simulink model "MicroMouseTemplate"  (R2024a)
settings: Solver=FixedStepAuto  StartTime=0.0  StopTime=10.0  RelTol=1e-3  EnableMultiTasking=on
undefined symbols (not defined in the file): DownLSThreshConv, DownRSThreshConv, FWDLSThreshConv, FWDRSThreshConv, LSThreshConv, RSThreshConv, samplingTime
settings Model: STM32="{\"DigitalPortWrite\":[{\"ID\":\"MicroMouseTemplate:84:10\"},{\"ID\":\"MicroMouseTemplate:84:9\"},{\"ID\":\"MicroMouseTemplate:84:8\"},{\"ID\":\"MicroMouseTemplate:84:7\"},{\"ID\":\"MicroMouseTemplate:84:6\"},{\"ID\":\"MicroMouseTemplate:84:5\"},{\"ID\":\"MicroMouseTemplate:84:4\"},{\"ID\":\"MicroMouseTemplate:84:3\"},{\"ID\":\"MicroMouseTemplate:160:19\"},{\"ID\":\"MicroMouseTemplate:2479:4\"},{\"ID\":\"MicroMouseTemplate:2479:6\"},{\"ID\":\"MicroMouseTemplate:2479:7\"},{\"ID\":\"MicroMouseTemplate:2479:8\"}],\"PWMOutput\":[{\"ID\":\"MicroMouseTemplate:160:24\"},{\"ID\":\"MicroMouseTemplate:160:25\"}],\"AnalogInput\":{\"ID\":\"MicroMouseTemplate:2357:1\"},\"DigitalPortRead\":[{\"ID\":\"MicroMouseTemplate:2483:3\"},{\"ID\":\"MicroMouseTemplate:2483:4\"}]}"  SimulationMode=external  ExtModeTrigDuration=10  Creator=JesseJabezArendse  LastModifiedBy=abdul
settings SolverCC: AllowMultiTaskInputOutput=on  AutoInsertRateTranBlk=on  InsertRTBMode=Never (minimum delay)
settings OptimizationCC: EnhancedBackFolding=on  PassReuseOutputArgsAs=Individual arguments  StateBitsets=on  DataBitsets=on  ZeroExternalMemoryAtStartup=off  ZeroInternalMemoryAtStartup=off  NoFixptDivByZeroProtection=on  MaxStackSize=64  OptimizeBlockOrder=speed  DifferentSizesBufferReuse=on  EfficientTunableParamExpr=on
settings DebuggingCC: MultiTaskCondExecSysMsg=none  ParameterOverflowMsg=none  ParameterPrecisionLossMsg=none  ParameterTunabilityLossMsg=error
settings HardwareCC: ProdBitPerPointer=32  ProdBitPerSizeT=32  ProdBitPerPtrDiffT=32  ProdLargestAtomicInteger=Long  ProdLargestAtomicFloat=Double  ProdWordSize=32  ProdLongLongMode=on  ProdHWDeviceType=ARM Compatible->ARM Cortex  TargetBitPerPointer=64  TargetBitPerSizeT=64  TargetBitPerPtrDiffT=64  TargetLongLongMode=on  TargetIntDivRoundTo=Zero  TargetEndianess=LittleEndian  TargetWordSize=64  TargetHWDeviceType=MATLAB Host
settings ModelReferenceCC: EnableParallelModelReferenceBuilds=on  ParallelModelReferenceMATLABWorkerInit=Copy Base Workspace  SupportModelReferenceSimTargetCustomCode=on
settings SFSimCC: MATLABDynamicMemAlloc=off  SimHardwareAcceleration=native
settings RTWCC: Description=Embedded Coder  SystemTargetFile=ert.tlc  HardwareBoard=STM32L4xx Based  TLCOptions=-p0 -aInlineSetEventsForThisBaseRateFcn=TLC_FALSE -aSuppressMultiTaskScheduler=TLC_FALSE -aRateBasedStepFcn=1  TemplateMakefile=ert_default_tmf  Toolchain=GNU Tools for ARM Embedded Processors  CodeExecutionProfiling=on  CodeProfilingInstrumentation=coarse  GPUComputeCapability=3.5
settings RTWCC: CustomHeaderCode=|
  | #include "MicroMouseProgramming\Core\Inc\IMU.h"
  | #include "MicroMouseProgramming\Core\Inc\CustomWhile.h"
  | #include "MicroMouseProgramming\Core\Inc\Motors.h"
settings RTWCC: CustomInclude=|
  | MicroMouseProgramming\Core\Inc\
  | MicroMouseProgramming\Core\Src\
settings RTWCC: CustomSource=|
  | MicroMouseProgramming\Core\Src\IMU.c
  | MicroMouseProgramming\Core\Src\CustomWhile.c
  | MicroMouseProgramming\Core\Src\Motors.c
settings CodeAppCC: ForceParamTrailComments=on  IgnoreCustomStorageClasses=off  OperatorAnnotations=on  SimulinkDataObjDesc=on  SFDataObjDesc=on  InsertBlockDesc=on
settings ERTTargetCC: CodeReplacementLibrary=ARM Cortex-M  SupportNonFinite=off  SupportComplex=off  SupportContinuousTime=on  ExtModeTransport=3  ExtModeStaticAlloc=on  ExtModeStaticAllocSize=2048  ExtModeMexFile=ext_xcp  ExtModeIntrfLevel=Level2 - Open

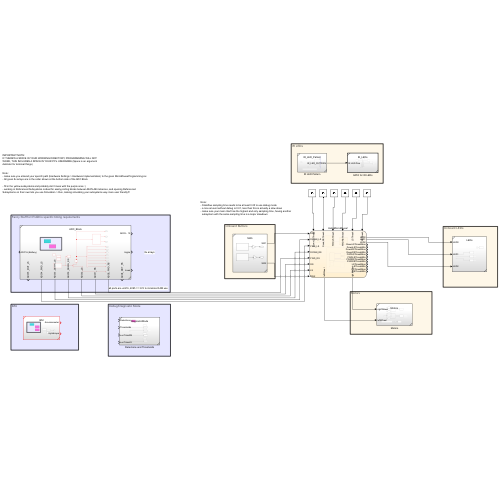
[thumbnail: Simulink's stored preview of the top-level diagram]
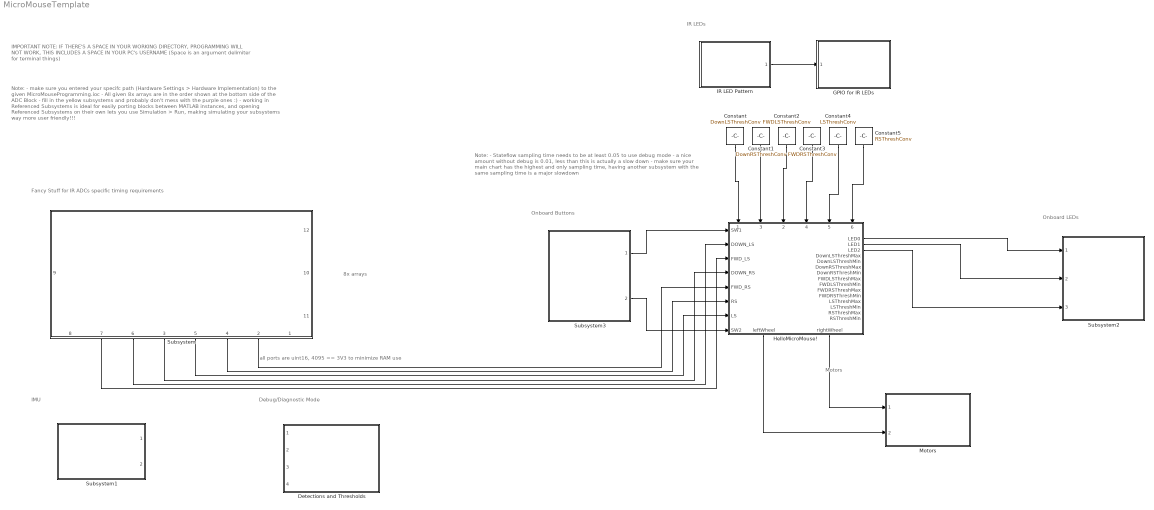
== system MicroMouseTemplate ==
  note: IMPORTANT NOTE:
      | IF THERE'S A SPACE IN YOUR WORKING DIRECTORY, PROGRAMMING WILL NOT WORK, THIS INCLUDES A SPACE IN YOUR PC's USERNAME (Space is an argument delimiter for terminal things)
  note: Note:
      | - make sure you entered your specifc path (Hardware Settings > Hardware Implementation) to the given MicroMouseProgramming.ioc
      | - All given 8x arrays are in the order shown at the bottom side of the ADC Block
      |
      | - fill in the yellow subsystems and probably don't mess with the purple ones :)
      | - working in Referenced Subsystems is ideal for easily porting blocks between MATLAB instances, and opening Referenced Subsystems on their own lets you use Simulation > Run, making simulating your subsystems way more user friendly!!!
  note: 8x arrays
  note: all ports are uint16, 4095 == 3V3 to minimize RAM use
  note: IMU
  note: Note:
      | - Stateflow sampling time needs to be at least 0.05 to use debug mode
      | - a nice amount without debug is 0.01, less than this is actually a slow down
      | - make sure your main chart has the highest and only sampling time, having another
      | subsystem with the same sampling time is a major slowdown
  note: Fancy Stuff for IR ADCs specific timing requirements
  note: IR LEDs
  note: Motors
  note: Onboard Buttons
  note: Onboard LEDs
  note: Debug/Diagnostic Mode
  Constant : Constant  Value=DownLSThreshConv
  Constant1 : Constant  Value=DownRSThreshConv
  Constant2 : Constant  Value=FWDLSThreshConv
  Constant3 : Constant  Value=FWDRSThreshConv
  Constant4 : Constant  Value=LSThreshConv
  Constant5 : Constant  Value=RSThreshConv
  Detections and Thresholds : Subsystem  ReferencedSubsystem=DiagnosticMode
  GPIO for IR LEDs : Subsystem  TreatAsAtomicUnit=on  SystemSampleTime=samplingTime  ReferencedSubsystem=IR_LEDs
  HelloMicroMouse! : Stateflow chart  TreatAsAtomicUnit=on
      settings: PortSchema="{\"entries\":[{\"content\":{\"sides\":[{\"content\":{\"connectorIds\":[\"In8\",\"In14\",\"In9\",\"In10\",\"In11\",\"In12\",\"In13\",\"In7\"]},\"type\":\"ConnectorPlacement.EquallySpacedRectSide\",\"uuid\":\"f52daa4f-6374-42e5-9ef1-0ccc99d09b58\"},{\"content\":{\"connectorIds\":[\"Out4\",\"Out1\",\"Out5\",\"Out6\",\"Out7\",\"Out8\",\"Out9\",\"Out10\",\"Out11\",\"Out12\",\"Out13\",\"Out14\",\"Out15\",\"Out16\",\"Out17\"],\"side\":\"RIGHT\"},\"type\":\"ConnectorPlacement.EquallySpacedRectSide\",\"uuid\":\"94b478cc-4dde-45c7-a588-77cf2b43cdb7\"},{\"content\":{\"connectorIds\":[\"In1\",\"In3\",\"In2\",\"In4\",\"In5\",\"In6\"],\"side\":\"TOP\"},\"type\":\"ConnectorPlacement.EquallySpacedRectSide\",\"uuid\":\"afff2079-ea5c-423e-9722-09c3bbce433b\"},{\"content\":{\"connectorIds\":[\"Out2\",\"Out3\"],\"side\":\"BOTTOM\"},\"type\":\"ConnectorPlacement.EquallySpacedRectSide\",\"uuid\":\"94e93a1d-795d-41a3-b2d8-d520b2bf47ef\"}]},\"type\":\"ConnectorPlacement.EquallySpacedConnector\",\"uuid\":\"d4d35636-54af-48ac-af70-d56caef5e090\"}],\"packageUris\":[\"http://schema.mathworks.com/mf0/Connector/R2020b\"],\"version\":\"1.0\"}"
  IR LED Pattern : Subsystem  ReferencedSubsystem=IR_LED_Pattern
  Motors : Subsystem  ReferencedSubsystem=Motors
  Subsystem : Subsystem  ReferencedSubsystem=ADC_Block
      settings: PortSchema="{\"entries\":[{\"content\":{\"sides\":[{\"content\":{},\"type\":\"ConnectorPlacement.EquallySpacedRectSide\",\"uuid\":\"be6b81d5-7a49-4e34-b35f-0c07892094fc\"},{\"content\":{\"connectorIds\":[\"Out1\",\"Out2\",\"Out4\",\"Out5\",\"Out3\",\"Out6\",\"Out7\",\"Out8\"],\"side\":\"RIGHT\"},\"type\":\"ConnectorPlacement.EquallySpacedRectSide\",\"uuid\":\"5e22590a-b7c0-4c63-8de4-8d81fd6c3849\"},{\"content\":{\"connectorIds\":[\"Out12\",\"Out10\",\"Out11\"],\"side\":\"TOP\"},\"type\":\"ConnectorPlacement.EquallySpacedRectSide\",\"uuid\":\"da97636e-cea0-4a10-8fe5-d807f9ee999f\"},{\"content\":{\"connectorIds\":[\"Out9\"],\"side\":\"BOTTOM\"},\"type\":\"ConnectorPlacement.EquallySpacedRectSide\",\"uuid\":\"a593d780-81a8-4730-a8bc-2bbf356cafe4\"}]},\"type\":\"ConnectorPlacement.EquallySpacedConnector\",\"uuid\":\"0bcac921-e51a-4437-9183-315712d0a8c2\"}],\"packageUris\":[\"http://schema.mathworks.com/mf0/Connector/R2020b\"],\"version\":\"1.0\"}"
  Subsystem1 : Subsystem  ReferencedSubsystem=IMU
  Subsystem2 : Subsystem  ReferencedSubsystem=LEDs
  Subsystem3 : Subsystem  ReferencedSubsystem=SWs
  wires:
  HelloMicroMouse!/2(leftWheel) -> Motors/2
  HelloMicroMouse!/3(rightWheel) -> Motors/1
  Subsystem3/1 -> HelloMicroMouse!/8(SW1)
  Subsystem3/2 -> HelloMicroMouse!/7(SW2)
  IR LED Pattern/1 -> GPIO for IR LEDs/1
  HelloMicroMouse!/1(LED1) -> Subsystem2/2
  HelloMicroMouse!/5(LED2) -> Subsystem2/3
  HelloMicroMouse!/4(LED0) -> Subsystem2/1
  Subsystem/6 -> HelloMicroMouse!/14(DOWN_LS)
  Constant/1 -> HelloMicroMouse!/1(DownLSThresh)
  Subsystem/3 -> HelloMicroMouse!/10(DOWN_RS)
  Subsystem/7 -> HelloMicroMouse!/9(FWD_LS)
  Subsystem/2 -> HelloMicroMouse!/11(FWD_RS)
  Subsystem/5 -> HelloMicroMouse!/13(LS)
  Subsystem/4 -> HelloMicroMouse!/12(RS)
  Constant1/1 -> HelloMicroMouse!/3(DownRSThresh)
  Constant2/1 -> HelloMicroMouse!/2(FWDLSThresh)
  Constant3/1 -> HelloMicroMouse!/4(FWDRSThresh)
  Constant4/1 -> HelloMicroMouse!/5(LSThresh)
  Constant5/1 -> HelloMicroMouse!/6(RSThresh)

== stateflow chart MicroMouseTemplate/HelloMicroMouse! ==
  state Calibration
    %--------------------
    entry:
    LED1 = true;
    rightWheel = 75;
    leftWheel = -75;
    % Meausure min/max voltage received
    DownLSThreshMin = DOWN_LS;
    DownRSThreshMin = DOWN_RS;
    FWDLSThreshMin = FWD_LS;
    FWDRSThreshMin = FWD_RS;
    LSThreshMin = LS;
    RSThreshMin = RS;
    DownLSThreshMax = DOWN_LS;
    DownRSThreshMax = DOWN_RS;
    FWDLSThreshMax = FWD_LS;
    FWDRSThreshMax = FWD_RS;
    LSThreshMax = LS;
    RSThreshMax = RS;
    %----------------------
    during:
    DownLSThreshMin = min([DownLSThresh, DOWN_LS]);
    DownRSThreshMin = min([DownRSThresh, DOWN_RS]);
    FWDLSThreshMin = min([FWDLSThresh, FWD_LS]);
    FWDRSThreshMin = min([FWDRSThresh, FWD_RS]);
    LSThreshMin = min([LSThresh, LS]);
    RSThreshMin = min([RSThresh, RS]);
    DownLSThreshMax = max([DownLSThresh, DOWN_LS]);
    DownRSThreshMax = max([DownRSThresh, DOWN_RS]);
    FWDLSThreshMax = max([FWDLSThresh, FWD_LS]);
    FWDRSThreshMax = max([FWDRSThresh, FWD_RS]);
    LSThreshMax = max([LSThresh, LS]);
    RSThreshMax = max([RSThresh, RS])
  state Calibrated
    %-----------------
    entry:
    rightWheel = 0;
    leftWheel = 0;
    LED0 = true;
    LED1 = true;
    LED2 = true;
    % Average threshold values
    DownLSThresh = mean([DownLSThreshMin, DownLSThreshMax]);
    DownRSThresh = mean([DownRSThreshMin, DownRSThreshMax]);
    FWDLSThresh = mean([FWDLSThreshMin, DownLSThreshMax]);
    FWDRSThresh = mean([FWDRSThreshMin, DownRSThreshMax]);
    LSThresh = mean([LSThreshMin, LSThreshMax]);
    RSThresh = mean([RSThreshMin, RSThreshMax]);
    % Set speed modes
    minSpeed = 75;
    medSpeed = 100;
    maxSpeed = 125;
  state WaitUntilButtonPressed
    during:
    LED0 = false;
    LED1 = ~LED1;
    LED2 = false;
    rightWheel = 0;
    leftWheel = 0;
  state On
    entry:
    LED0 = false;
    LED1 = true;
    LED2 = false;
    exit:
    leftWheel = 0;
    rightWheel = 0;
    state Forward
      during:
      rightWheel = min;
      leftWheel= min;
      exit:
      rightWheel = min;
      leftWheel= min;
    state WadeLeft
      during:
      LED0 = true;
      rightWheel = rightWheel + 2;
      leftWheel = leftWheel + 3;
      exit:
      LED0 = false;
    state Slow
      during:
      LED0 = true;
      LED2 = true;
      rightWheel = rightWheel - 10;
      leftWheel = leftWheel - 10;
      exit:
      LED0 = false;
      LED2 = false;
    state WadeRight
      during:
      LED2 = true;
      rightWheel = rightWheel + 3;
      leftWheel = leftWheel + 2;
      exit:
      LED2 = false;
    state TurnRight [commented out]
      during:
      rightWheel = rightWheel;
      leftWheel = leftWheel + 10;
      LED2 = ~LED2;
      exit:
      LED2 = false;
    state TurnLeft [commented out]
      during:
      rightWheel = rightWheel +10;
      leftWheel = leftWheel;
      LED0 = ~LED0;
      exit:
      LED0 = false;
    (default) -> Forward
    Forward -> WadeLeft [order 2] : [DOWN_RS > DownRSThresh]
    WadeLeft -> Forward [order 1] : [DOWN_RS < DownRSThresh]
    WadeLeft -> Slow [order 2] : [FWD_LS > FWDLSThresh]
    WadeRight -> WadeLeft [order 3] : [DOWN_RS > DownRSThresh]
    WadeLeft -> WadeRight [order 3] : [DOWN_LS > DownLSThresh]
    Forward -> WadeRight [order 1] : [DOWN_LS > DownLSThresh]
    WadeRight -> Forward [order 2] : [DOWN_LS < DownLSThresh]
    WadeRight -> Slow [order 1] : [FWD_RS > FWDRSThresh]
    Forward -> Slow [order 3] : [FWD_LS > FWDLSThresh || FWD_RS > FWDRSThresh]
    (junction 156) -> Forward : [FWD_RS < FWDRSThresh]
    TurnRight -> Forward [commented out] : [FWD_LS < FWDLSThresh]
    Slow -> (junction 160) [order 2]
    Slow -> (junction 164) [order 1] : [LS < LSThresh ]
    (junction 160) -> (junction 158) : [RS < RSThresh]
    (junction 158) -> TurnRight [commented out]
    (junction 164) -> TurnLeft [commented out] : [LS < LSThresh ]
    TurnLeft -> (junction 156) [commented out] : [FWD_RS < FWDRSThresh]
  (default) -> WaitUntilButtonPressed
  WaitUntilButtonPressed -> Calibration : [SW1]
  Calibration -> ? : [SW2]
  Calibration -> Calibrated [order 1] : after(5, sec)
  Calibrated -> On : [SW1]
  data: DownLSThresh input; FWDLSThresh input; DownRSThresh input; FWDRSThresh input; LSThresh input; RSThresh input; SW2 input; LED1 output; SW1 input; FWD_LS input; DOWN_RS input; FWD_RS input; RS input; LS input; leftWheel output int8; rightWheel output int8; LED0 output; LED2 output; DOWN_LS input; DownLSThreshMax output; DownLSThreshMin output; DownRSThreshMax output; DownRSThreshMin output; FWDLSThreshMax output; FWDLSThreshMin output; FWDRSThreshMax output; FWDRSThreshMin output; LSThreshMax output; LSThreshMin output; RSThreshMax output; RSThreshMin output; minSpeed local; medSpeed local; maxSpeed local
